simulink model "Stewart"  (R2016a)
settings: Solver=FixedStepAuto  StartTime=0.0  StopTime=inf  RelTol=1e-3
libraries: arduinolib x18, neural x6, simulink x1
settings Model: SimulationMode=external  ExtModeTrigDuration=2  Creator=costa  LastModifiedBy=costa
settings OptimizationCC: OptimizeModelRefInitCode=on  LifeSpan=1  MaxStackSize=64
settings HardwareCC: ProdBitPerInt=16  ProdBitPerPointer=16  ProdLargestAtomicFloat=None  ProdWordSize=8  ProdHWDeviceType=Atmel->AVR
settings RTWCC: SystemTargetFile=ert.tlc  HardwareBoard=Arduino Mega 2560  TemplateMakefile=ert_default_tmf  GenerateReport=on  Toolchain=Arduino AVR v1.6.1  BuildConfiguration=Faster Runs  IncludeHyperlinkInReport=on  LaunchReport=on  GenerateTraceInfo=on  GenerateTraceReport=on  GenerateTraceReportSl=on  GenerateTraceReportSf=on  GenerateTraceReportEml=on
settings CodeAppCC: ForceParamTrailComments=on  IgnoreCustomStorageClasses=off  OperatorAnnotations=on  SimulinkDataObjDesc=on  SFDataObjDesc=on  MATLABFcnDesc=on  MangleLength=10  InsertBlockDesc=on  MATLABSourceComments=on
settings ERTTargetCC: SupportContinuousTime=on  SupportVariableSizeSignals=on  ExtMode=on  ExtModeTransport=3  ExtModeMexFile=ext_serial_win32_comm_rtt  ExtModeMexArgs=0 5 115200

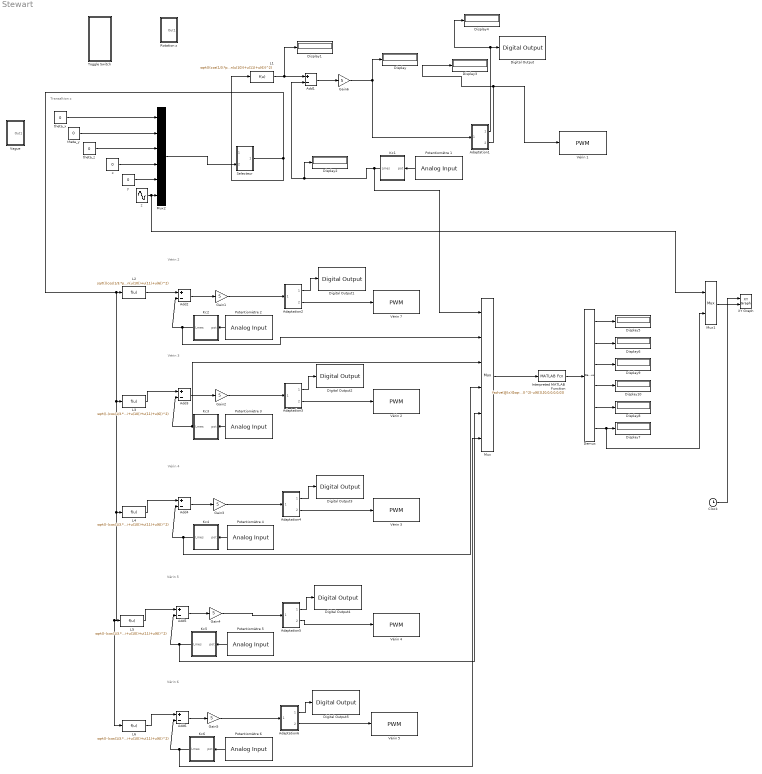
== system Stewart ==
  note: Transaltion z
  note: Vérin 6
  note: Vérin 5
  note: Vérin 4
  note: Vérin 3
  note: Vérin 2
  Adaptation1 : Subsystem
  Adaptation2 : Subsystem
  Adaptation3 : Subsystem
  Adaptation4 : Subsystem
  Adaptation5 : Subsystem
  Adaptation6 : Subsystem
  Add{1..6} (6 alike) : Sum  Inputs=+-
  Clock : Clock
  Demux : Demux  Outputs=6
  Digital Output : arduinolib/Digital Output  pinNumber=11  blockPlatform=arduino
  Digital Output1 : arduinolib/Digital Output  pinNumber=5  blockPlatform=arduino
  Digital Output2 : arduinolib/Digital Output  pinNumber=3  blockPlatform=arduino
  Digital Output3 : arduinolib/Digital Output  pinNumber=9  blockPlatform=arduino
  Digital Output4 : arduinolib/Digital Output  pinNumber=7  blockPlatform=arduino
  Digital Output5 : arduinolib/Digital Output  pinNumber=13  blockPlatform=arduino
  Display{,1..10} (11 alike) : Display
  Gain{1..6} (6 alike) : Gain  Gain=5
  Interpreted MATLAB Function : MATLABFcn  MATLABFcn=fsolve(@(x)([sqrt(((cos(1/3.*pi+x(3))*cos(x(2))-sin(1/3.*pi+x(3))*sin(x(1))*sin(x(2)))*rm*cos(beta)+sin(1/3.*pi+x(3))*cos(x(1))*rm*sin(beta)-rf*cos(alpha)+x(4))^2+ ((sin(1/3.*pi+x(3))*cos(x(2))+cos(1/3.*pi+x(3))*sin(x(1))*sin(x(2)))*rm*cos(beta)-cos(1/3.*pi+x(3))*cos(x(1))*rm*sin(beta)-rf*sin(alpha)+x(5))^2+ (-cos(x(1))*sin(x(2))*rm*cos(beta)-sin(x(1))*rm*sin(beta)+h+x(6))^2)-u(1),sqrt(((cos(1/3.*pi+x(3))*cos(x(2))-sin(1/3.*pi+x(3))*sin(x(1))*sin(x(2)))*rm*cos(beta)-sin(1/3.*pi+x(3))*cos(x(1))*rm*sin(beta)+rf*cos(1/3.*pi+alpha)+x(4))^2+ ((sin(1/3.*pi+x(3))*cos(x(2))+cos(1/3.*pi+x(3))*sin(x(1))*sin(x(2)))*rm*cos(beta)+cos(1/3.*pi+x(3))*cos(x(1))*rm*sin(beta)-rf*sin(1/3.*pi+alpha)+x(5))^2+ (-cos(x(1))*sin(x(2))*rm*cos(beta)+sin(x(1))*rm*sin(beta)+h+x(6))^2)-u(2),sqrt((-(cos(1/3.*pi+x(3))*cos(x(2))-sin(1/3.*pi+x(3))*sin(x(1))*sin(x(2)))*rm*cos(1/3.*pi+beta)-sin(1/3.*pi+x(3))*cos(x(1))*rm*sin(1/3.*pi+beta)+rf*sin(1/6.*pi+alpha)+x(4))^2+(-(sin(1/3.*pi+x(3))*cos(x(2))+cos(1/3.*pi+x(3))*sin(x(1))*sin(x(2)))*rm*cos(1/3.*pi+beta)+cos(1/3.*pi+x(3))*cos(x(1))*rm*sin(1/3.*pi+beta)-rf*cos(1/6.*pi+alpha)+x(5))^2+(cos(x(1))*sin(x(2))*rm*cos(1/3.*pi+beta)+sin(x(1))*rm*sin(1/3.*pi+beta)+h+x(6))^2)-u(3),sqrt((-(cos(1/3.*pi+x(3))*cos(x(2))-sin(1/3.*pi+x(3))*sin(x(1))*sin(x(2)))*rm*sin(1/6.*pi+beta)-sin(1/3.*pi+x(3))*cos(x(1))*rm*cos(1/6.*pi+beta)+rf*sin(1/6.*pi+alpha)+x(4))^2+(-(sin(1/3.*pi+x(3))*cos(x(2))+cos(1/3.*pi+x(3))*sin(x(1))*sin(x(2)))*rm*sin(1/6.*pi+beta)+cos(1/3.*pi+x(3))*cos(x(1))*rm*cos(1/6.*pi+beta)+rf*cos(1/6.*pi+alpha)+x(5))^2+(cos(x(1))*sin(x(2))*rm*sin(1/6.*pi+beta)+sin(x(1))*rm*cos(1/6.*pi+beta)+h+x(6))^2)-u(4),sqrt((-(cos(1/3.*pi+x(3))*cos(x(2))-sin(1/3.*pi+x(3))*sin(x(1))*sin(x(2)))*rm*sin(1/6.*pi+beta)+sin(1/3.*pi+x(3))*cos(x(1))*rm*cos(1/6.*pi+beta)+rf*cos(1/3.*pi+alpha)+x(4))^2+(-(sin(1/3.*pi+x(3))*cos(x(2))+cos(1/3.*pi+x(3))*sin(x(1))*sin(x(2)))*rm*sin(1/6.*pi+beta)-cos(1/3.*pi+x(3))*cos(x(1))*rm*cos(1/6.*pi+beta)+rf*sin(1/3.*pi+alpha)+x(5))^2+(cos(x(1))*sin(x(2))*rm*sin(1/6.*pi+beta)-sin(x(1))*rm*cos(1/6.*pi+beta)+h+x(6))^2)-u(5),sqrt((-(cos(1/3.*pi+x(3))*cos(x(2))-sin(1/3.*pi+x(3))*sin(x(1))*sin(x(2)))*rm*cos(1/3.*pi+beta)+sin(1/3.*pi+x(3))*cos(x(1))*rm*sin(1/3.*pi+beta)-rf*cos(alpha)+x(4))^2+(-(sin(1/3.*pi+x(3))*cos(x(2))+cos(1/3.*pi+x(3))*sin(x(1))*sin(x(2)))*rm*cos(1/3.*pi+beta)-cos(1/3.*pi+x(3))*cos(x(1))*rm*sin(1/3.*pi+beta)+rf*sin(alpha)+x(5))^2+(cos(x(1))*sin(x(2))*rm*cos(1/3.*pi+beta)-sin(x(1))*rm*sin(1/3.*pi+beta)+h+x(6))^2)-u(6)]),[0,0,0,0,0,0])  OutputDimensions=6
  Kc1 : Subsystem
  Kc2 : Subsystem
  Kc3 : Subsystem
  Kc4 : Subsystem
  Kc5 : Subsystem
  Kc6 : Subsystem
  L1 : Fcn  Expr=sqrt(((cos(1/3.*pi+u(3))*cos(u(2))-sin(1/3.*pi+u(3))*sin(u(1))*sin(u(2)))*u(7)*cos(u(10))+sin(1/3.*pi+u(3))*cos(u(1))*u(7)*sin(u(10))-u(8)*cos(u(9))+u(4))^2+ ((sin(1/3.*pi+u(3))*cos(u(2))+cos(1/3.*pi+u(3))*sin(u(1))*sin(u(2)))*u(7)*cos(u(10))-cos(1/3.*pi+u(3))*cos(u(1))*u(7)*sin(u(10))-u(8)*sin(u(9))+u(5))^2+ (-cos(u(1))*sin(u(2))*u(7)*cos(u(10))-sin(u(1))*u(7)*sin(u(10))+u(11)+u(6))^2)
  L2 : Fcn  Expr=sqrt(((cos(1/3.*pi+u(3))*cos(u(2))-sin(1/3.*pi+u(3))*sin(u(1))*sin(u(2)))*u(7)*cos(u(10))-sin(1/3.*pi+u(3))*cos(u(1))*u(7)*sin(u(10))+u(8)*cos(1/3.*pi+u(9))+u(4))^2+ ((sin(1/3.*pi+u(3))*cos(u(2))+cos(1/3.*pi+u(3))*sin(u(1))*sin(u(2)))*u(7)*cos(u(10))+cos(1/3.*pi+u(3))*cos(u(1))*u(7)*sin(u(10))-u(8)*sin(1/3.*pi+u(9))+u(5))^2+ (-cos(u(1))*sin(u(2))*u(7)*cos(u(10))+sin(u(1))*u(7)*sin(u(10))+u(11)+u(6))^2)
  L3 : Fcn  Expr=sqrt((-(cos(1/3.*pi+u(3))*cos(u(2))-sin(1/3.*pi+u(3))*sin(u(1))*sin(u(2)))*u(7)*cos(1/3.*pi+u(10))-sin(1/3.*pi+u(3))*cos(u(1))*u(7)*sin(1/3.*pi+u(10))+u(8)*sin(1/6.*pi+u(9))+u(4))^2+(-(sin(1/3.*pi+u(3))*cos(u(2))+cos(1/3.*pi+u(3))*sin(u(1))*sin(u(2)))*u(7)*cos(1/3.*pi+u(10))+cos(1/3.*pi+u(3))*cos(u(1))*u(7)*sin(1/3.*pi+u(10))-u(8)*cos(1/6.*pi+u(9))+u(5))^2+(cos(u(1))*sin(u(2))*u(7)*cos(1/3.*pi+u(10))+sin(u(1))*u(7)*sin(1/3.*pi+u(10))+u(11)+u(6))^2)
  L4 : Fcn  Expr=sqrt((-(cos(1/3.*pi+u(3))*cos(u(2))-sin(1/3.*pi+u(3))*sin(u(1))*sin(u(2)))*u(7)*sin(1/6.*pi+u(10))-sin(1/3.*pi+u(3))*cos(u(1))*u(7)*cos(1/6.*pi+u(10))+u(8)*sin(1/6.*pi+u(9))+u(4))^2+(-(sin(1/3.*pi+u(3))*cos(u(2))+cos(1/3.*pi+u(3))*sin(u(1))*sin(u(2)))*u(7)*sin(1/6.*pi+u(10))+cos(1/3.*pi+u(3))*cos(u(1))*u(7)*cos(1/6.*pi+u(10))+u(8)*cos(1/6.*pi+u(9))+u(5))^2+(cos(u(1))*sin(u(2))*u(7)*sin(1/6.*pi+u(10))+sin(u(1))*u(7)*cos(1/6.*pi+u(10))+u(11)+u(6))^2)
  L5 : Fcn  Expr=sqrt((-(cos(1/3.*pi+u(3))*cos(u(2))-sin(1/3.*pi+u(3))*sin(u(1))*sin(u(2)))*u(7)*sin(1/6.*pi+u(10))+sin(1/3.*pi+u(3))*cos(u(1))*u(7)*cos(1/6.*pi+u(10))+u(8)*cos(1/3.*pi+u(9))+u(4))^2+(-(sin(1/3.*pi+u(3))*cos(u(2))+cos(1/3.*pi+u(3))*sin(u(1))*sin(u(2)))*u(7)*sin(1/6.*pi+u(10))-cos(1/3.*pi+u(3))*cos(u(1))*u(7)*cos(1/6.*pi+u(10))+u(8)*sin(1/3.*pi+u(9))+u(5))^2+(cos(u(1))*sin(u(2))*u(7)*sin(1/6.*pi+u(10))-sin(u(1))*u(7)*cos(1/6.*pi+u(10))+u(11)+u(6))^2)
  L6 : Fcn  Expr=sqrt((-(cos(1/3.*pi+u(3))*cos(u(2))-sin(1/3.*pi+u(3))*sin(u(1))*sin(u(2)))*u(7)*cos(1/3.*pi+u(10))+sin(1/3.*pi+u(3))*cos(u(1))*u(7)*sin(1/3.*pi+u(10))-u(8)*cos(u(9))+u(4))^2+(-(sin(1/3.*pi+u(3))*cos(u(2))+cos(1/3.*pi+u(3))*sin(u(1))*sin(u(2)))*u(7)*cos(1/3.*pi+u(10))-cos(1/3.*pi+u(3))*cos(u(1))*u(7)*sin(1/3.*pi+u(10))+u(8)*sin(u(9))+u(5))^2+(cos(u(1))*sin(u(2))*u(7)*cos(1/3.*pi+u(10))-sin(u(1))*u(7)*sin(1/3.*pi+u(10))+u(11)+u(6))^2)
  Mux : Mux  Inputs=6
  Mux1 : Mux  Inputs=2
  Mux2 : Mux  Inputs=6
  Potentiomètre 1 : arduinolib/Analog Input  pinNumber=2  sampleTime=0.001  blockPlatform=arduino
  Potentiomètre 2 : arduinolib/Analog Input  pinNumber=1  sampleTime=0.001  blockPlatform=arduino
  Potentiomètre 3 : arduinolib/Analog Input  pinNumber=0  sampleTime=0.001  blockPlatform=arduino
  Potentiomètre 4 : arduinolib/Analog Input  pinNumber=5  sampleTime=0.001  blockPlatform=arduino
  Potentiomètre 5 : arduinolib/Analog Input  pinNumber=4  sampleTime=0.001  blockPlatform=arduino
  Potentiomètre 6 : arduinolib/Analog Input  pinNumber=3  sampleTime=0.001  blockPlatform=arduino
  Rotation z : Subsystem
  Selecteur : Subsystem
  Toggle Switch : Subsystem  DialogController=hmiCreateDDGDialog  IsWebBlock=on  mask(MWDashboardBlock){webBlockId=66615d0e-4370-4182-87d5-3900dd51e72f, webBlockType=toggleswitch, ShowInLibBrowser=on, ShowInitialText=on, HMISrcModelName=Stewart}
      mask prompts: webBlockId "WebBlock Id"; webBlockType "WebBlock Type"; HMISrcModelName "Source Model"
      mask Help: helpview([docroot '/mapfiles/simulink.map'], 'hmi_toggle_switch')
      mask Display:
      | if strcmp(get_param(bdroot(gcb),'BlockDiagramType'), 'library')
      |     image([(matlabroot) '/toolbox/simulink/hmi/icons/ToggleSwitch.png']);
      | end
  Vague : Subsystem
  Vérin 1 : arduinolib/PWM  pinNumber=10  blockPlatform=arduino
  Vérin 2 : arduinolib/PWM  pinNumber=2  blockPlatform=arduino
  Vérin 3 : arduinolib/PWM  pinNumber=8  blockPlatform=arduino
  Vérin 4 : arduinolib/PWM  pinNumber=6  blockPlatform=arduino
  Vérin 5 : arduinolib/PWM  pinNumber=12  blockPlatform=arduino
  Vérin 7 : arduinolib/PWM  pinNumber=4  blockPlatform=arduino
  XY Graph : simulink/Sinks/XY Graph  xmin=0  xmax=10  ymin=0  ymax=600  st=-1
  theta_x : Constant  Value=0
  theta_y : Constant  Value=0
  theta_z : Constant  Value=0
  x : Constant  Value=0
  y : Constant  Value=0
  z : Sin  Amplitude=50  Frequency=60  SampleTime=0
  wires:
  Potentiomètre 1/1 -> Kc1/1(pot)
  L1/1 -> Display1/1, Add1/1
  Gain6/1 -> Display/1, Adaptation1/1(ecart)
  Adaptation1/1(sens) -> Display4/1, Digital Output/1
  Adaptation1/2(pwm) -> Display3/1, Vérin 1/1
  Add1/1 -> Gain6/1
  Clock/1 -> XY Graph/1
  Selecteur/1(Out1) -> L6/1, L5/1, L4/1, L3/1, L2/1, L1/1
  Mux2/1 -> Selecteur/2(In2)
  Gain1/1 -> Adaptation2/1(ecart)
  L2/1 -> Add2/1
  Adaptation2/1(sens) -> Digital Output1/1
  Adaptation2/2(pwm) -> Vérin 7/1
  Potentiomètre 2/1 -> Kc2/1(pot)
  Add2/1 -> Gain1/1
  Kc2/1(Lmes) -> Mux/2, Add2/2
  L3/1 -> Add3/1
  Adaptation3/1(sens) -> Digital Output2/1
  Adaptation3/2(pwm) -> Vérin 2/1
  Gain2/1 -> Adaptation3/1(ecart)
  Add3/1 -> Gain2/1
  Potentiomètre 3/1 -> Kc3/1(pot)
  L4/1 -> Add4/1
  Gain3/1 -> Adaptation4/1(ecart)
  Adaptation4/1(sens) -> Digital Output3/1
  Adaptation4/2(pwm) -> Vérin 3/1
  Kc4/1(Lmes) -> Mux/4, Add4/2
  Potentiomètre 4/1 -> Kc4/1(pot)
  Add4/1 -> Gain3/1
  L5/1 -> Add5/1
  Adaptation5/1(sens1) -> Digital Output4/1
  Adaptation5/2(pwm1) -> Vérin 4/1
  Potentiomètre 5/1 -> Kc5/1(pot)
  Add5/1 -> Gain4/1
  Kc5/1(Lmes) -> Mux/5, Add5/2
  Gain4/1 -> Adaptation5/1(ecart1)
  L6/1 -> Add6/1
  Adaptation6/1(sens) -> Digital Output5/1
  Adaptation6/2(pwm) -> Vérin 5/1
  Potentiomètre 6/1 -> Kc6/1(pot)
  Kc6/1(Lmes) -> Mux/6, Add6/2
  Add6/1 -> Gain5/1
  Gain5/1 -> Adaptation6/1(ecart)
  Kc1/1(Lmes) -> Mux/1, Display2/1, Add1/2
  Kc3/1(Lmes) -> Add3/2, Mux/3
  Mux/1 -> Interpreted MATLAB Function/1
  Interpreted MATLAB Function/1 -> Demux/1
  Demux/1 -> Display5/1
  Demux/2 -> Display6/1
  Demux/3 -> Display9/1
  Demux/4 -> Display10/1
  Demux/5 -> Display8/1
  Demux/6 -> Mux1/2, Display7/1
  Mux1/1 -> XY Graph/2
  z/1 -> Mux1/1, Mux2/6
  x/1 -> Mux2/4
  theta_x/1 -> Mux2/1
  y/1 -> Mux2/5
  theta_z/1 -> Mux2/3
  theta_y/1 -> Mux2/2

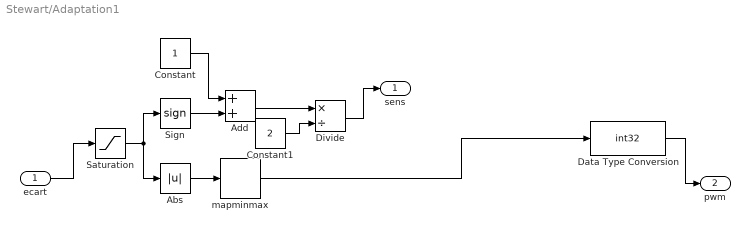
== system Stewart/Adaptation1 ==
  ecart : Inport
  Abs : Abs
  Add : Sum
  Constant : Constant
  Constant1 : Constant  Value=2
  Data Type Conversion : DataTypeConversion  OutDataTypeStr=int32
  Divide : Product  Inputs=*/
  Saturation : Saturate  UpperLimit=200  LowerLimit=-200
  Sign : Signum
  mapminmax : neural/Processing Functions/mapminmax  xmin=0  xmax=200  ymin=1  ymax=255
  sens : Outport
  pwm : Outport  Port=2
  wires:
  ecart/1 -> Saturation/1
  Abs/1 -> mapminmax/1
  Saturation/1 -> Sign/1, Abs/1
  Sign/1 -> Add/2
  Constant/1 -> Add/1
  Add/1 -> Divide/1
  Constant1/1 -> Divide/2
  Divide/1 -> sens/1
  Data Type Conversion/1 -> pwm/1
  mapminmax/1 -> Data Type Conversion/1

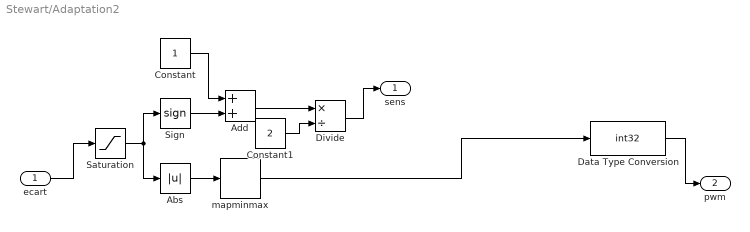
== system Stewart/Adaptation2 ==
  ecart : Inport
  Abs : Abs
  Add : Sum
  Constant : Constant
  Constant1 : Constant  Value=2
  Data Type Conversion : DataTypeConversion  OutDataTypeStr=int32
  Divide : Product  Inputs=*/
  Saturation : Saturate  UpperLimit=200  LowerLimit=-200
  Sign : Signum
  mapminmax : neural/Processing Functions/mapminmax  xmin=0  xmax=200  ymin=1  ymax=255
  sens : Outport
  pwm : Outport  Port=2
  wires:
  ecart/1 -> Saturation/1
  Abs/1 -> mapminmax/1
  Saturation/1 -> Sign/1, Abs/1
  Sign/1 -> Add/2
  Constant/1 -> Add/1
  Add/1 -> Divide/1
  Constant1/1 -> Divide/2
  Divide/1 -> sens/1
  Data Type Conversion/1 -> pwm/1
  mapminmax/1 -> Data Type Conversion/1

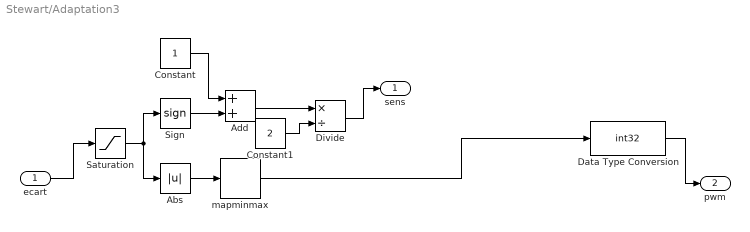
== system Stewart/Adaptation3 ==
  ecart : Inport
  Abs : Abs
  Add : Sum
  Constant : Constant
  Constant1 : Constant  Value=2
  Data Type Conversion : DataTypeConversion  OutDataTypeStr=int32
  Divide : Product  Inputs=*/
  Saturation : Saturate  UpperLimit=200  LowerLimit=-200
  Sign : Signum
  mapminmax : neural/Processing Functions/mapminmax  xmin=0  xmax=200  ymin=1  ymax=255
  sens : Outport
  pwm : Outport  Port=2
  wires:
  ecart/1 -> Saturation/1
  Abs/1 -> mapminmax/1
  Saturation/1 -> Sign/1, Abs/1
  Sign/1 -> Add/2
  Constant/1 -> Add/1
  Add/1 -> Divide/1
  Constant1/1 -> Divide/2
  Divide/1 -> sens/1
  Data Type Conversion/1 -> pwm/1
  mapminmax/1 -> Data Type Conversion/1

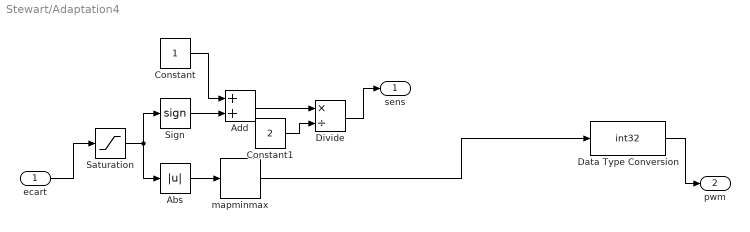
== system Stewart/Adaptation4 ==
  ecart : Inport
  Abs : Abs
  Add : Sum
  Constant : Constant
  Constant1 : Constant  Value=2
  Data Type Conversion : DataTypeConversion  OutDataTypeStr=int32
  Divide : Product  Inputs=*/
  Saturation : Saturate  UpperLimit=200  LowerLimit=-200
  Sign : Signum
  mapminmax : neural/Processing Functions/mapminmax  xmin=0  xmax=200  ymin=1  ymax=255
  sens : Outport
  pwm : Outport  Port=2
  wires:
  ecart/1 -> Saturation/1
  Abs/1 -> mapminmax/1
  Saturation/1 -> Sign/1, Abs/1
  Sign/1 -> Add/2
  Constant/1 -> Add/1
  Add/1 -> Divide/1
  Constant1/1 -> Divide/2
  Divide/1 -> sens/1
  Data Type Conversion/1 -> pwm/1
  mapminmax/1 -> Data Type Conversion/1

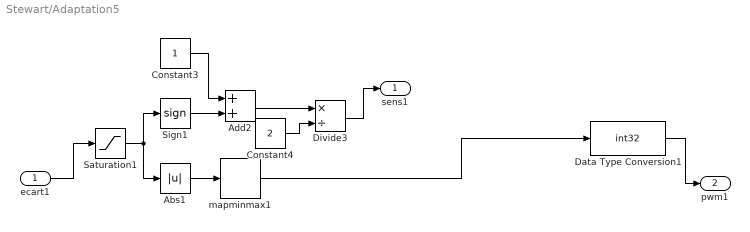
== system Stewart/Adaptation5 ==
  ecart1 : Inport
  Abs1 : Abs
  Add2 : Sum
  Constant3 : Constant
  Constant4 : Constant  Value=2
  Data Type Conversion1 : DataTypeConversion  OutDataTypeStr=int32
  Divide3 : Product  Inputs=*/
  Saturation1 : Saturate  UpperLimit=200  LowerLimit=-200
  Sign1 : Signum
  mapminmax1 : neural/Processing Functions/mapminmax  xmin=0  xmax=200  ymin=1  ymax=255
  sens1 : Outport
  pwm1 : Outport  Port=2
  wires:
  ecart1/1 -> Saturation1/1
  Abs1/1 -> mapminmax1/1
  Saturation1/1 -> Sign1/1, Abs1/1
  Sign1/1 -> Add2/2
  Constant3/1 -> Add2/1
  Add2/1 -> Divide3/1
  Constant4/1 -> Divide3/2
  Divide3/1 -> sens1/1
  Data Type Conversion1/1 -> pwm1/1
  mapminmax1/1 -> Data Type Conversion1/1

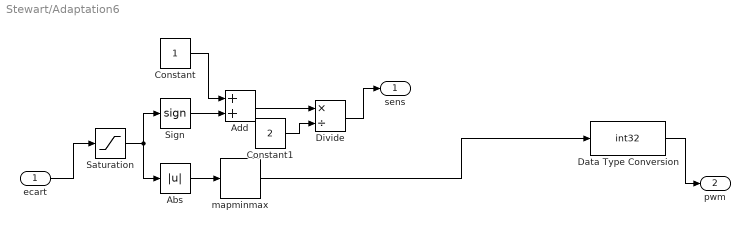
== system Stewart/Adaptation6 ==
  ecart : Inport
  Abs : Abs
  Add : Sum
  Constant : Constant
  Constant1 : Constant  Value=2
  Data Type Conversion : DataTypeConversion  OutDataTypeStr=int32
  Divide : Product  Inputs=*/
  Saturation : Saturate  UpperLimit=200  LowerLimit=-200
  Sign : Signum
  mapminmax : neural/Processing Functions/mapminmax  xmin=0  xmax=200  ymin=1  ymax=255
  sens : Outport
  pwm : Outport  Port=2
  wires:
  ecart/1 -> Saturation/1
  Abs/1 -> mapminmax/1
  Saturation/1 -> Sign/1, Abs/1
  Sign/1 -> Add/2
  Constant/1 -> Add/1
  Add/1 -> Divide/1
  Constant1/1 -> Divide/2
  Divide/1 -> sens/1
  Data Type Conversion/1 -> pwm/1
  mapminmax/1 -> Data Type Conversion/1

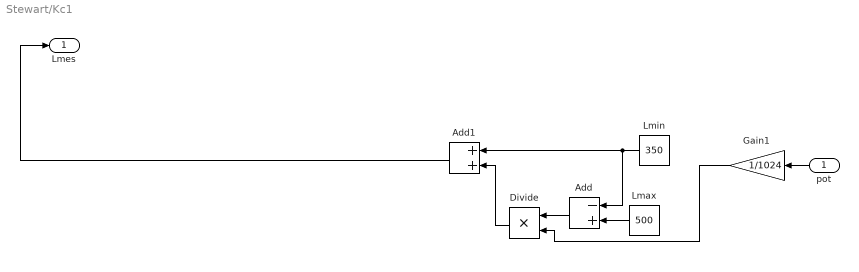
== system Stewart/Kc1 ==
  pot : Inport
  Add : Sum  Inputs=-+
  Add1 : Sum
  Divide : Product  Inputs=**
  Gain1 : Gain  Gain=1/1024
  Lmax : Constant  Value=500
  Lmin : Constant  Value=350
  Lmes : Outport
  wires:
  Lmin/1 -> Add1/1, Add/1
  Lmax/1 -> Add/2
  Gain1/1 -> Divide/2
  Divide/1 -> Add1/2
  Add1/1 -> Lmes/1
  pot/1 -> Gain1/1
  Add/1 -> Divide/1

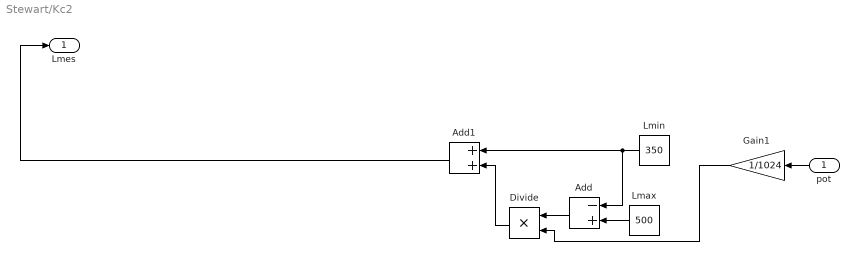
== system Stewart/Kc2 ==
  pot : Inport
  Add : Sum  Inputs=-+
  Add1 : Sum
  Divide : Product  Inputs=**
  Gain1 : Gain  Gain=1/1024
  Lmax : Constant  Value=500
  Lmin : Constant  Value=350
  Lmes : Outport
  wires:
  Lmin/1 -> Add1/1, Add/1
  Lmax/1 -> Add/2
  Gain1/1 -> Divide/2
  Divide/1 -> Add1/2
  Add1/1 -> Lmes/1
  pot/1 -> Gain1/1
  Add/1 -> Divide/1

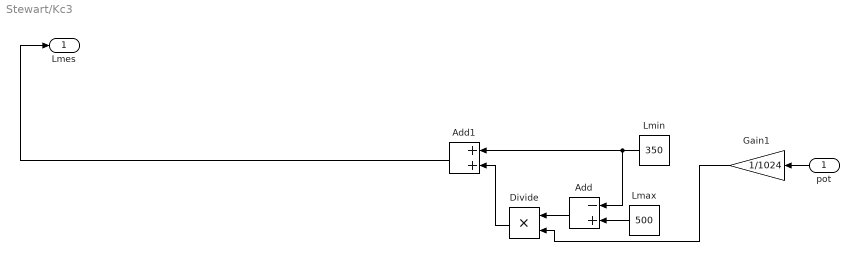
== system Stewart/Kc3 ==
  pot : Inport
  Add : Sum  Inputs=-+
  Add1 : Sum
  Divide : Product  Inputs=**
  Gain1 : Gain  Gain=1/1024
  Lmax : Constant  Value=500
  Lmin : Constant  Value=350
  Lmes : Outport
  wires:
  Lmin/1 -> Add1/1, Add/1
  Lmax/1 -> Add/2
  Gain1/1 -> Divide/2
  Divide/1 -> Add1/2
  Add1/1 -> Lmes/1
  pot/1 -> Gain1/1
  Add/1 -> Divide/1

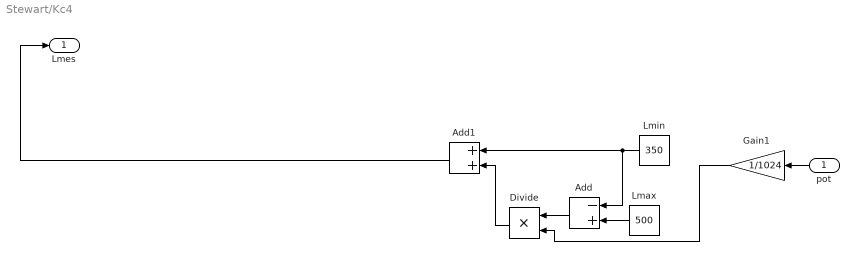
== system Stewart/Kc4 ==
  pot : Inport
  Add : Sum  Inputs=-+
  Add1 : Sum
  Divide : Product  Inputs=**
  Gain1 : Gain  Gain=1/1024
  Lmax : Constant  Value=500
  Lmin : Constant  Value=350
  Lmes : Outport
  wires:
  Lmin/1 -> Add1/1, Add/1
  Lmax/1 -> Add/2
  Gain1/1 -> Divide/2
  Divide/1 -> Add1/2
  Add1/1 -> Lmes/1
  pot/1 -> Gain1/1
  Add/1 -> Divide/1

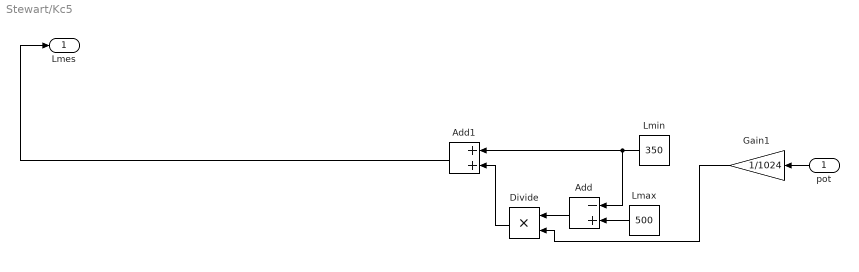
== system Stewart/Kc5 ==
  pot : Inport
  Add : Sum  Inputs=-+
  Add1 : Sum
  Divide : Product  Inputs=**
  Gain1 : Gain  Gain=1/1024
  Lmax : Constant  Value=500
  Lmin : Constant  Value=350
  Lmes : Outport
  wires:
  Lmin/1 -> Add1/1, Add/1
  Lmax/1 -> Add/2
  Gain1/1 -> Divide/2
  Divide/1 -> Add1/2
  Add1/1 -> Lmes/1
  pot/1 -> Gain1/1
  Add/1 -> Divide/1

== system Stewart/Kc6 ==
  pot : Inport
  Add : Sum  Inputs=-+
  Add1 : Sum
  Divide : Product  Inputs=**
  Gain1 : Gain  Gain=1/1024
  Lmax : Constant  Value=500
  Lmin : Constant  Value=350
  Lmes : Outport
  wires:
  Lmin/1 -> Add1/1, Add/1
  Lmax/1 -> Add/2
  Gain1/1 -> Divide/2
  Divide/1 -> Add1/2
  Add1/1 -> Lmes/1
  pot/1 -> Gain1/1
  Add/1 -> Divide/1

== system Stewart/Rotation z ==
  Mux1 : Mux  Inputs=6
  theta_x : Constant  Value=0
  theta_y : Constant  Value=0
  theta_z : Sin  Amplitude=pi/8  Frequency=40  SampleTime=0
  x : Constant  Value=0
  y : Constant  Value=0
  z : Constant  Value=0
  Out1 : Outport
  wires:
  theta_y/1 -> Mux1/2
  theta_z/1 -> Mux1/3
  y/1 -> Mux1/5
  theta_x/1 -> Mux1/1
  x/1 -> Mux1/4
  z/1 -> Mux1/6
  Mux1/1 -> Out1/1

== system Stewart/Selecteur ==
  In1 : Inport
  In2 : Inport  Port=2
  Mux : Mux  Inputs=2
  Paramètres mécanisme : Subsystem
  Stop : Subsystem
  Switch : Switch  Threshold=-1
  Out1 : Outport
  wires:
  Paramètres mécanisme/1(Out1) -> Mux/2
  In1/1 -> Switch/2
  In2/1 -> Switch/3
  Switch/1 -> Mux/1
  Mux/1 -> Out1/1
  Stop/1(Out1) -> Switch/1

== system Stewart/Toggle Switch ==

== system Stewart/Vague ==
  Mux1 : Mux  Inputs=6
  theta_x : Sin  Amplitude=pi/8  Frequency=40  SampleTime=0
  theta_y : Sin  Amplitude=pi/8  Frequency=40  Phase=pi/2  SampleTime=0
  theta_z : Constant  Value=0
  x : Constant  Value=0
  y : Constant  Value=0
  z : Constant  Value=0
  Out1 : Outport
  wires:
  theta_y/1 -> Mux1/2
  theta_z/1 -> Mux1/3
  y/1 -> Mux1/5
  theta_x/1 -> Mux1/1
  x/1 -> Mux1/4
  z/1 -> Mux1/6
  Mux1/1 -> Out1/1

== system Stewart/Selecteur/Paramètres mécanisme ==
  Mux1 : Mux  Inputs=5
  alpha : Constant  Value=0.007
  beta : Constant  Value=0.009
  h : Constant  Value=380
  rf : Constant  Value=270
  rm : Constant  Value=200
  Out1 : Outport
  wires:
  Mux1/1 -> Out1/1
  rm/1 -> Mux1/1
  rf/1 -> Mux1/2
  alpha/1 -> Mux1/3
  beta/1 -> Mux1/4
  h/1 -> Mux1/5

== system Stewart/Selecteur/Stop ==
  Mux1 : Mux  Inputs=6
  theta_x : Constant  Value=0
  theta_y : Constant  Value=0
  theta_z : Constant  Value=0
  x : Constant  Value=0
  y : Constant  Value=0
  z : Constant  Value=0
  Out1 : Outport
  wires:
  theta_y/1 -> Mux1/2
  theta_z/1 -> Mux1/3
  y/1 -> Mux1/5
  theta_x/1 -> Mux1/1
  x/1 -> Mux1/4
  z/1 -> Mux1/6
  Mux1/1 -> Out1/1
